simulink model "FM_recv_Cordic"  (R2019a)
settings: Solver=VariableStepAuto  StartTime=0.0  StopTime=0.1  RelTol=1e-3
libraries: dspfdesign x4, commanapbnd3 x2
settings Model: Creator=Wunyje  LastModifiedBy=Wunyje

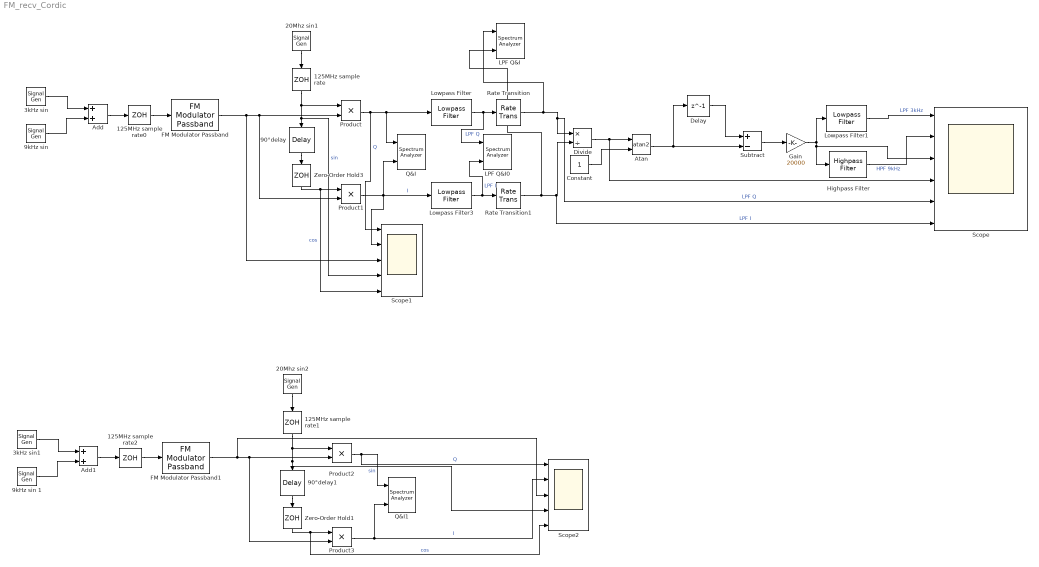
== system FM_recv_Cordic ==
  125MHz sample rate : ZeroOrderHold  SampleTime=8E-9
  125MHz sample rate0 : ZeroOrderHold  SampleTime=8e-9
  125MHz sample rate1 : ZeroOrderHold  SampleTime=4E-9
  125MHz sample rate2 : ZeroOrderHold  SampleTime=4e-9
  20Mhz sin1 : SignalGenerator  Frequency=20e6
  20Mhz sin2 : SignalGenerator  Frequency=20e6
  3kHz sin : SignalGenerator  Frequency=3000
  3kHz sin1 : SignalGenerator  Frequency=3000
  90°delay : TransportDelay  DelayTime=12.5e-9
  90°delay1 : TransportDelay  DelayTime=12.5e-9
  "9kHz sin " : SignalGenerator  Frequency=9000
  9kHz sin 1 : SignalGenerator  Frequency=9000
  Add : Sum
  Add1 : Sum
  Atan : Trigonometry  Operator=atan2  ApproximationMethod=CORDIC  NumberOfIterations=15
  Constant : Constant  OutDataTypeStr=fixdt(1,16,14)  SampleTime=5e-6
  Delay : Delay  DelayLength=1  InitialCondition=0
  Divide : Product  Inputs=*/  OutMin=0  OutMax=0.06  OutDataTypeStr=fixdt(1,16,14)
  FM Modulator Passband : commanapbnd3/FM Modulator Passband  Fc=20e6  Ph=0  Kc=50
      settings: SourceProductName=Communications Toolbox  SourceProductBaseCode=CM
  FM Modulator Passband1 : commanapbnd3/FM Modulator Passband  Fc=20e6  Ph=0  Kc=50
      settings: SourceProductName=Communications Toolbox  SourceProductBaseCode=CM
  Gain : Gain  Gain=20000
  Highpass Filter : dspfdesign/Highpass Filter  FilterType=FIR  DesignForMinimumOrder=on  FilterOrder=50  StopbandFrequency=4e3  PassbandFrequency=6e3  StopbandAttenuation=80  PassbandRipple=0.1  InheritSampleRate=off  SampleRate=200e3  SimulateUsing=Interpreted execution  roundingMode=Floor  coeffsDataTypeStr=fixdt(1,16)
      settings: SourceProductName=DSP System Toolbox
  LPF Q&I : SpectrumAnalyzer  NumInputPorts=2
  LPF Q&I0 : SpectrumAnalyzer  NumInputPorts=2
  Lowpass Filter : dspfdesign/Lowpass Filter  FilterType=FIR  DesignForMinimumOrder=on  FilterOrder=50  PassbandFrequency=2e6  StopbandFrequency=3e6  PassbandRipple=0.1  StopbandAttenuation=180  InheritSampleRate=off  SampleRate=125e6  SimulateUsing=Interpreted execution  roundingMode=Floor  coeffsDataTypeStr=fixdt(1,16)
  Lowpass Filter1 : dspfdesign/Lowpass Filter  FilterType=FIR  DesignForMinimumOrder=on  FilterOrder=50  PassbandFrequency=5e3  StopbandFrequency=7e3  PassbandRipple=0.1  StopbandAttenuation=80  InheritSampleRate=off  SampleRate=200e3  SimulateUsing=Interpreted execution  roundingMode=Floor  coeffsDataTypeStr=fixdt(1,16)
  Lowpass Filter3 : dspfdesign/Lowpass Filter  FilterType=FIR  DesignForMinimumOrder=on  FilterOrder=50  PassbandFrequency=2e6  StopbandFrequency=3e6  PassbandRipple=0.1  StopbandAttenuation=180  InheritSampleRate=on  SampleRate=200e3  SimulateUsing=Interpreted execution  roundingMode=Floor  coeffsDataTypeStr=fixdt(1,16)
  Product{,1..3} (4 alike) : Product
  Q&I : SpectrumAnalyzer  NumInputPorts=2
  Q&I1 : SpectrumAnalyzer  NumInputPorts=2
  Rate Transition : RateTransition  OutPortSampleTimeOpt=Multiple of input port sample time  OutPortSampleTimeMultiple=625
  Rate Transition1 : RateTransition  OutPortSampleTimeOpt=Multiple of input port sample time  OutPortSampleTimeMultiple=625
  Scope : Scope  NumInputPorts=6
  Scope1 : Scope  NumInputPorts=5
  Scope2 : Scope  NumInputPorts=5
  Subtract : Sum  Inputs=+-
  Zero-Order Hold1 : ZeroOrderHold  SampleTime=4E-9
  Zero-Order Hold3 : ZeroOrderHold  SampleTime=8E-9
  wires:
  90°delay/1 -> Zero-Order Hold3/1
  Zero-Order Hold3/1 -> Scope1/5, Product1/1  "cos"
  Product/1 -> Scope1/1, Q&I/1, Lowpass Filter/1  "Q"
  20Mhz sin1/1 -> 125MHz sample rate/1
  Subtract/1 -> Gain/1
  Lowpass Filter1/1 -> Scope/1  "LPF 3kHz"
  Atan/1 -> Subtract/2, Delay/1
  Rate Transition1/1 -> LPF Q&I/2, Scope/6, Divide/2  "LPF I"
  Gain/1 -> Highpass Filter/1, Scope/3, Lowpass Filter1/1
  Add/1 -> 125MHz sample rate0/1
  Highpass Filter/1 -> Scope/2  "HPF 9kHz"
  Product1/1 -> Scope1/2, Q&I/2, Lowpass Filter3/1  "I"
  Lowpass Filter/1 -> LPF Q&I0/1, Rate Transition/1  "LPF Q"
  "9kHz sin "/1 -> Add/2
  Delay/1 -> Subtract/1
  125MHz sample rate/1 -> Scope1/4, 90°delay/1, Product/1  "sin"
  Rate Transition/1 -> LPF Q&I/1, Scope/5, Divide/1  "LPF Q"
  125MHz sample rate0/1 -> FM Modulator Passband/1
  Lowpass Filter3/1 -> LPF Q&I0/2, Rate Transition1/1  "LPF I"
  3kHz sin/1 -> Add/1
  Divide/1 -> Atan/1, Scope/4
  Constant/1 -> Atan/2
  FM Modulator Passband/1 -> Scope1/3, Product/2, Product1/2
  90°delay1/1 -> Zero-Order Hold1/1
  20Mhz sin2/1 -> 125MHz sample rate1/1
  125MHz sample rate1/1 -> Scope2/4, 90°delay1/1, Product2/1  "sin"
  9kHz sin 1/1 -> Add1/2
  FM Modulator Passband1/1 -> Scope2/3, Product2/2, Product3/2
  Zero-Order Hold1/1 -> Scope2/5, Product3/1  "cos"
  3kHz sin1/1 -> Add1/1
  Product3/1 -> Scope2/2, Q&I1/2  "I"
  Add1/1 -> 125MHz sample rate2/1
  Product2/1 -> Scope2/1, Q&I1/1  "Q"
  125MHz sample rate2/1 -> FM Modulator Passband1/1
